simulink model "simulation"  (R2024a)
settings: Solver=VariableStepAuto  StartTime=0.0  StopTime=50  RelTol=1e-3
undefined symbols (not defined in the file): k, T
settings Model: Creator=paulhondola  LastModifiedBy=paulhondola

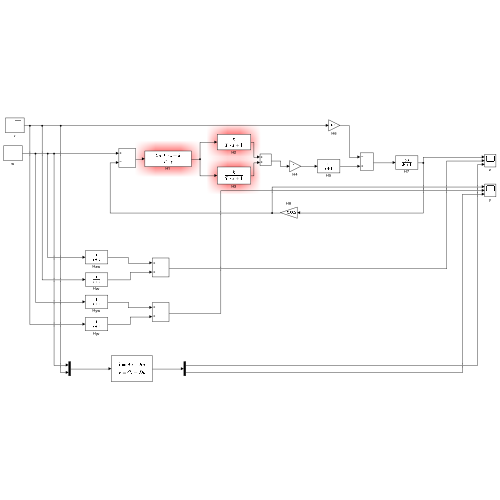
[thumbnail: Simulink's stored preview of the top-level diagram]
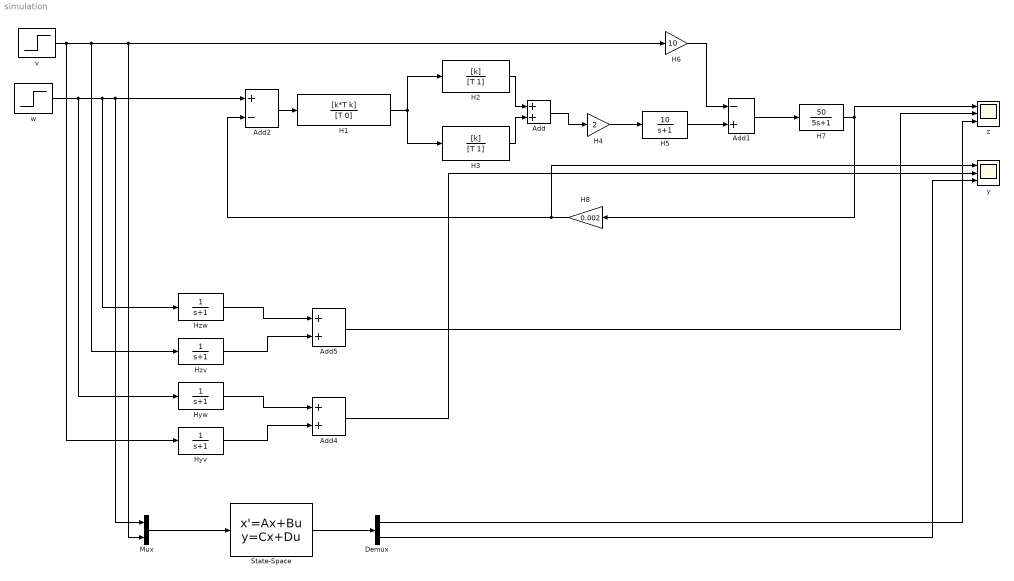
== system simulation ==
  Add : Sum
  Add1 : Sum  Inputs=-+
  Add2 : Sum  Inputs=+-
  Add4 : Sum
  Add5 : Sum
  Demux : Demux  Outputs=2
  H1 : TransferFcn  Numerator=[k*T k]  Denominator=[T 0]
  H2 : TransferFcn  Numerator=[k]  Denominator=[T 1]
  H3 : TransferFcn  Numerator=[k]  Denominator=[T 1]
  H4 : Gain  Gain=2
  H5 : TransferFcn  Numerator=[10]  Denominator=[1 1]
  H6 : Gain  Gain=10
  H7 : TransferFcn  Numerator=[50]  Denominator=[5 1]
  H8 : Gain  Gain=0.002
  Hyv : TransferFcn  Denominator=[1 1]
  Hyw : TransferFcn  Denominator=[1 1]
  Hzv : TransferFcn  Denominator=[1 1]
  Hzw : TransferFcn  Denominator=[1 1]
  Mux : Mux  Inputs=2
  State-Space : StateSpace  InitialCondition=0
  v : Step  Time=25  SampleTime=0
  w : Step  Time=0  After=5  SampleTime=0
  y : Scope  NumInputPorts=3
  z : Scope  NumInputPorts=3
  wires:
  H2/1 -> Add/1
  H3/1 -> Add/2
  Add/1 -> H4/1
  H4/1 -> H5/1
  H1/1 -> H3/1, H2/1
  v/1 -> Hyv/1, Hzv/1, Mux/2, H6/1
  H6/1 -> Add1/1
  Add1/1 -> H7/1
  H7/1 -> z/1, H8/1
  Add2/1 -> H1/1
  w/1 -> Hyw/1, Hzw/1, Mux/1, Add2/1
  H8/1 -> y/1, Add2/2
  H5/1 -> Add1/2
  Hyw/1 -> Add4/1
  Hyv/1 -> Add4/2
  Hzw/1 -> Add5/1
  Hzv/1 -> Add5/2
  Add5/1 -> z/2
  Add4/1 -> y/2
  Mux/1 -> State-Space/1
  State-Space/1 -> Demux/1
  Demux/1 -> z/3
  Demux/2 -> y/3
